simulink library "hose_pump_unit_v3"  (R2024a)
settings: Solver=VariableStepAuto  StartTime=0.0  StopTime=10.0  RelTol=1e-3
undefined symbols (not defined in the file): fiber_angle_alpha, fiber_angle_alpha_unstr, hose_pump_max_stretch, HP_spring_stiffness, HP_stretched_radius, HP_unstretched_length, HP_unstretched_radius, Lt, mu, regulator_set_pressure_PSI, Rt
libraries: fl_lib x5, nesl_utility x4, SimscapeFluids_lib x2
settings Model: Creator=Carson  LastModifiedBy=Carson

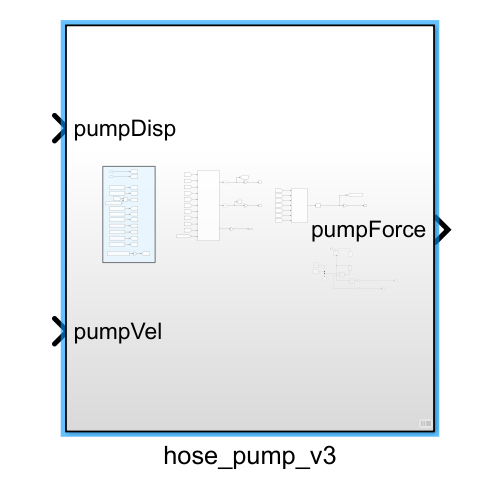
[thumbnail: Simulink's stored preview of the top-level diagram]
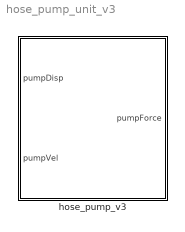
== system hose_pump_unit_v3 ==
  hose_pump_v3 : Subsystem

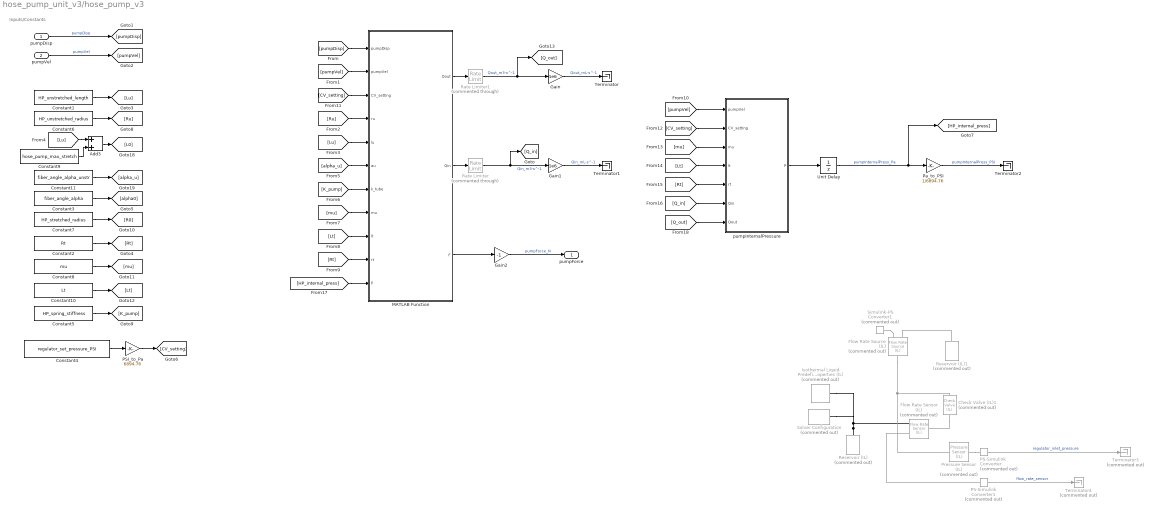
== system hose_pump_unit_v3/hose_pump_v3 ==
  note: Inputs/Constants
  pumpDisp : Inport
  pumpVel : Inport  Port=2
  Add3 : Sum
  Check Valve (IL)1 : SimscapeFluids_lib/Isothermal Liquid/Valves & Orifices/Directional Control Valves/Check Valve (IL)  Commented=on  opening_spec=fluids.isothermal_liquid.valves_orifices.enum.PressureOpeningSpec.Linear  pressure_control_spec=fluids.isothermal_liquid.valves_orifices.enum.pressure_control_spec.dp  p_crack_differential=regulator_set_pressure_PSI psi  p_crack_gauge=0.1 MPa  press_max_differential=regulator_set_pressure_PSI+1 psi  press_max_gauge=0.2 MPa  area_max=1e-4 m^2  area_leak=1e-10 m^2  p_diff_TLU=[0.01 : 0.01 : 0.1] MPa  valve_area_TLU=[1e-10, 1e-05, 2e-05, 3e-05, 4e-05, 5e-05, 6e-05, 7.5e-05, 8.5e-05, .0001] m^2  vol_flow_TLU=[.000358, .045, .11, .191, .284, .39, .505, .63, .764, .905] .* 1e-3 m^3/s  area=inf m^2  Cd=0.64  Re_c=150  smoothing_factor=0.01  pressure_recovery=false  opening_dynamics=false  tau=0.1 s  enable_faults=simscape.enum.onoff.off  fault_action=fluids.enum.FaultOpening.Closed
      settings: InternalSimscapePortConfiguration="{\"Bottom\":[],\"Left\":[{\"id\":\"A\",\"label\":\"A\",\"type\":\"foundation.isothermal_liquid.isothermal_liquid\"}],\"Right\":[{\"id\":\"B\",\"label\":\"B\",\"type\":\"foundation.isothermal_liquid.isothermal_liquid\"}],\"Top\":[]}"
  Constant1 : Constant  Value=HP_unstretched_length
  Constant10 : Constant  Value=Lt
  Constant11 : Constant  Value=fiber_angle_alpha_unstr
  Constant2 : Constant  Value=Rt
  Constant3 : Constant  Value=fiber_angle_alpha
  Constant4 : Constant  Value=regulator_set_pressure_PSI
  Constant5 : Constant  Value=HP_spring_stiffness
  Constant6 : Constant  Value=HP_unstretched_radius
  Constant7 : Constant  Value=HP_stretched_radius
  Constant8 : Constant  Value=mu
  Constant9 : Constant  Value=hose_pump_max_stretch
  Flow Rate Sensor (IL) : fl_lib/Isothermal Liquid/Sensors/Flow Rate Sensor (IL)  Commented=on  sensor_type=foundation.enum.mass_volumetric_sensor.volumetric
      settings: InternalSimscapePortConfiguration="{\"Bottom\":[],\"Left\":[{\"id\":\"A\",\"label\":\"A\",\"type\":\"foundation.isothermal_liquid.isothermal_liquid\"}],\"Right\":[{\"id\":\"B\",\"label\":\"B\",\"type\":\"foundation.isothermal_liquid.isothermal_liquid\"},{\"id\":\"V\",\"label\":\"V\",\"type\":\"output\"}],\"Top\":[]}"
  Flow Rate Source (IL) : fl_lib/Isothermal Liquid/Sources/Flow Rate Source (IL)  Commented=on  source_type=foundation.enum.constant_controlled.controlled  flow_type=foundation.enum.mass_volumetric_flow.volumetric  mass_flow=0 kg/s  volumetric_flow=0 m^3/s
      settings: InternalSimscapePortConfiguration="{\"Bottom\":[],\"Left\":[{\"id\":\"A\",\"label\":\"A\",\"type\":\"foundation.isothermal_liquid.isothermal_liquid\"},{\"id\":\"V\",\"label\":\"V\",\"type\":\"input\"}],\"Right\":[{\"id\":\"B\",\"label\":\"B\",\"type\":\"foundation.isothermal_liquid.isothermal_liquid\"}],\"Top\":[]}"
  Gain : Gain  Gain=1e6
  Gain1 : Gain  Gain=1e6
  Gain2 : Gain  Gain=-1
  Isothermal Liquid Predefined Properties (IL) : SimscapeFluids_lib/Isothermal Liquid/Utilities/Isothermal Liquid Predefined Properties (IL)  Commented=on  fluid_list=fluids.isothermal_liquid.utilities.enum.isothermal_liquid_fluid_list.water  concentration_param_EG=fluids.isothermal_liquid.utilities.enum.isothermal_liquid_concentration.volume_fraction  concentration_param_PG=fluids.isothermal_liquid.utilities.enum.isothermal_liquid_concentration.volume_fraction  c_mass_SW=3.5e-3  c_mass_EG=0.1  c_mass_PG=0.1  c_mass_GL=0.1  c_vol_EG=0.1  c_vol_PG=0.1  beta_L_atm_EG=2.1791 GPa  beta_L_atm_PG=2.1791 GPa  beta_L_atm_GL=2.1791 GPa  p_min_EG=0.01 MPa  p_min_PG=0.01 MPa  p_min_GL=0.01 MPa  T=293.15 K  derate_coeff=1  p_atm=0.101325 MPa  properties_range_check=simscape.enum.assert.action.warn  air_fraction=0  polytropic_index=1.0  rho_g_atm=1.225 kg/m^3  air_dissolution_model=false  p_crit=3 MPa
      settings: InternalSimscapePortConfiguration="{\"Bottom\":[],\"Left\":[],\"Right\":[{\"id\":\"A\",\"label\":\"\",\"type\":\"foundation.isothermal_liquid.isothermal_liquid\"}],\"Top\":[]}"
  MATLAB Function : MATLAB Function  TreatAsAtomicUnit=on
  PS-Simulink Converter : nesl_utility/PS-Simulink Converter  Commented=on  PhysicalDomain=network_engine_domain  SubClassName=ps_output  LeftPortType=input  RightPortType=output  PseudoPeriodic=off  Frequencies=[]  VectorFormat=inherit  Unit=Pa  AffineConversion=off
  PS-Simulink Converter1 : nesl_utility/PS-Simulink Converter  Commented=on  PhysicalDomain=network_engine_domain  SubClassName=ps_output  LeftPortType=input  RightPortType=output  PseudoPeriodic=off  Frequencies=[]  VectorFormat=inherit  Unit=m^3/s  AffineConversion=off
  PSI_to_Pa : Gain  Gain=6894.76
  Pa_to_PSI : Gain  Gain=1/6894.76
  Pressure Sensor (IL) : fl_lib/Isothermal Liquid/Sensors/Pressure Sensor (IL)  Commented=on  pressure_measure=foundation.enum.pressure_measure.gauge
      settings: InternalSimscapePortConfiguration="{\"Bottom\":[],\"Left\":[{\"id\":\"A\",\"label\":\"A\",\"type\":\"foundation.isothermal_liquid.isothermal_liquid\"}],\"Right\":[{\"id\":\"Pg\",\"label\":\"Pg\",\"type\":\"output\"}],\"Top\":[]}"
  Rate Limiter : RateLimiter  Commented=through  RisingSlewLimit=1e-3  FallingSlewLimit=-1e-3  SampleTimeMode=inherited
  Rate Limiter1 : RateLimiter  Commented=through  RisingSlewLimit=1e-3  FallingSlewLimit=-1e-3  SampleTimeMode=inherited
  Reservoir (IL) : fl_lib/Isothermal Liquid/Elements/Reservoir (IL)  Commented=on  reservoir_type=foundation.enum.constant_controlled.constant  pressure_spec=foundation.enum.pressure_spec.atmospheric  reservoir_pressure=0.101325 MPa
  Reservoir (IL)1 : fl_lib/Isothermal Liquid/Elements/Reservoir (IL)  Commented=on  reservoir_type=foundation.enum.constant_controlled.constant  pressure_spec=foundation.enum.pressure_spec.atmospheric  reservoir_pressure=0.101325 MPa
  Simulink-PS Converter1 : nesl_utility/Simulink-PS Converter  Commented=on  PhysicalDomain=network_engine_domain  SubClassName=ps_input  LeftPortType=input  RightPortType=output  PseudoPeriodic=off  Frequencies=[]  NoiseDistribution=none  NoiseParameters=[]  Unit=m^3/s  AffineConversion=off  FilteringAndDerivatives=zero  SimscapeFilterOrder=1  InputFilterTimeConstant=0.001  UdotUserProvided=0
  Solver Configuration : nesl_utility/Solver Configuration  Commented=on  PhysicalDomain=network_engine_domain  SubClassName=solver  LeftPortType=input  RightPortType=generic  Tones=[]  Harmonics=[]  SimulateNoise=off  Profile=off  UseLocalSampling=off  EnableSwitchedLinearOptims=on  FrequencyDomain=off  UseCCode=off  RelTol=0.001  AbsTol=1e-06  MinStep=1e-09  ToWorkspace=off  RevertToSquareIcSolve=off  NumHomotopyIterations=100  PhasorMode=off  PhasorModeNumHarmonics=1  ConsistencySolver=NEWTON_XTOL_AFTER_FTOL  IndexReductionMethod=DerivativeReplacement  DoDC=on  ResidualTolerance=1e-09  ConsistencyTolSource=GLOBAL  ConsistencyAbsTol=0.001  ConsistencyRelTol=0.001  ConsistencyTolFactor=0.001  UseLocalSolver=on  LocalSolverChoice=NE_BACKWARD_EULER_ADVANCER  ResolveIndetEquations=on  FunctionEvalNumThread=1  LocalSolverSampleTime=simu.dt  DoFixedCost=off  MaxNonlinIter=3  MaxModeIter=2  ComputeImpulses=off  ImpulseIterations=2  LinearAlgebra=auto  LinearAlgebraNumThread=0  EquationFormulation=NE_TIME_EF  DelaysMemoryBudget=1024  AutomaticFiltering=off  FilteringTimeConstant=0.001  PartitionStorageMethod=AS_NEEDED  PartitionMemoryBudget=1024  PartitionMethod=FAST  MultibodyUseLocalSolver=off  MultibodyLocalSolverChoice=ODE1  MultibodyLocalSolverSampleTime=0.001
  Terminator : Terminator
  Terminator1 : Terminator
  Terminator2 : Terminator
  Terminator3 : Terminator  Commented=on
  Terminator4 : Terminator  Commented=on
  Unit Delay : UnitDelay  SampleTime=-1  HasFrameUpgradeWarning=on
  pumpInternalPressure : MATLAB Function  TreatAsAtomicUnit=on
  pumpForce : Outport
  wires:
  Constant3/1 -> [alpha0]
  Constant2/1 -> [Rt]
  Constant1/1 -> [Lu]
  Constant5/1 -> [K_pump]
  Constant9/1 -> Add3/2
  [Lu] -> Add3/1
  Add3/1 -> [L0]
  Constant11/1 -> [alpha_u]
  pumpDisp/1 -> [pumpDisp]  "pumpDisp"
  pumpVel/1 -> [pumpVel]  "pumpVel"
  Constant6/1 -> [Ru]
  Constant7/1 -> [R0]
  Constant8/1 -> [mu]
  Constant10/1 -> [Lt]
  [pumpDisp] -> MATLAB Function/1(pumpDisp)
  [pumpVel] -> MATLAB Function/2(pumpVel)
  [Ru] -> MATLAB Function/4(ru)
  [Lu] -> MATLAB Function/5(lu)
  [alpha_u] -> MATLAB Function/6(au)
  [K_pump] -> MATLAB Function/7(k_tube)
  [mu] -> MATLAB Function/8(mu)
  [Lt] -> MATLAB Function/9(lt)
  [Rt] -> MATLAB Function/10(rt)
  Rate Limiter1/1 -> [Q_out], Gain/1  "Qout_m3-s^-1"
  Rate Limiter/1 -> [Q_in], Gain1/1  "Qin_m3-s^-1"
  Unit Delay/1 -> [HP_internal_press], Pa_to_PSI/1  "pumpInternalPress_Pa"
  [CV_setting] -> MATLAB Function/3(CV_setting)
  Gain/1 -> Terminator/1  "Qout_mL-s^-1"
  Gain1/1 -> Terminator1/1  "Qin_mL-s^-1"
  Pa_to_PSI/1 -> Terminator2/1  "pumpInternalPress_PSI"
  Gain2/1 -> pumpForce/1  "pumpForce_N"
  MATLAB Function/3(F) -> Gain2/1
  [pumpVel] -> pumpInternalPressure/1(pumpVel)
  Constant4/1 -> PSI_to_Pa/1
  PSI_to_Pa/1 -> [CV_setting]
  [CV_setting] -> pumpInternalPressure/2(CV_setting)
  [mu] -> pumpInternalPressure/3(mu)
  [Lt] -> pumpInternalPressure/4(lt)
  [Rt] -> pumpInternalPressure/5(rt)
  [Q_in] -> pumpInternalPressure/6(Qin)
  [HP_internal_press] -> MATLAB Function/11(P)
  pumpInternalPressure/1(P) -> Unit Delay/1
  PS-Simulink Converter/1 -> Terminator3/1  "regulator_inlet_pressure"
  PS-Simulink Converter1/1 -> Terminator4/1  "flow_rate_sensor"
  [Q_out] -> pumpInternalPressure/7(Qout)
  MATLAB Function/2(Qin) -> Rate Limiter/1
  MATLAB Function/1(Qout) -> Rate Limiter1/1
  connections:
  Reservoir (IL)/LConn1 -- Flow Rate Sensor (IL)/RConn1 -- Solver Configuration/RConn1 -- Isothermal Liquid Predefined Properties (IL)/RConn1
  Flow Rate Source (IL)/RConn1 -- Check Valve (IL)1/LConn1 -- Pressure Sensor (IL)/LConn1
  PS-Simulink Converter1/LConn1 -- Flow Rate Sensor (IL)/RConn2
  Reservoir (IL)1/LConn1 -- Flow Rate Source (IL)/LConn1
  Simulink-PS Converter1/RConn1 -- Flow Rate Source (IL)/LConn2
  Check Valve (IL)1/RConn1 -- Flow Rate Sensor (IL)/LConn1
  Pressure Sensor (IL)/RConn1 -- PS-Simulink Converter/LConn1

== matlab function hose_pump_unit_v3/hose_pump_v3/MATLAB Function ==
  data: pumpDisp input; pumpVel input; CV_setting input; Qout output; ru input; lu input; au input; k_tube input; mu input; lt input; rt input; Qin output; F output; P input
function [Qout, Qin, F] = pumpDisplacementCalcs(pumpDisp, pumpVel, CV_setting, ru, lu, au, k_tube, mu, lt, rt, P)

if pumpVel > 0 % pumping water out
    % P = CV_setting; % assume internal pressure immediately rises to check valve set pressure
    % F = pi * ru^2 * P * (3 * (pumpDisp/lu+1)^2 / (tan(au))^2 - 1/sin(au)^2) + k_tube*pumpDisp;
    Qout = -pi * ru^2 * (1/sin(au)^2 - 3 * (pumpDisp/lu+1)^2 / (tan(au))^2) * pumpVel;
    Qin = 0;
else
    % F = k_tube*pumpDisp;
    Qin = pi * ru^2 * (1/sin(au)^2 - 3 * (pumpDisp/lu+1)^2 / (tan(au))^2) * pumpVel;
    Qout = 0;
    % P = -8*mu*lt/(pi*rt^4)*Qin;
end

F = pi * ru^2 * max([P, 0]) * (3 * (pumpDisp/lu+1)^2 / (tan(au))^2 - 1/sin(au)^2) + k_tube*pumpDisp;

== matlab function hose_pump_unit_v3/hose_pump_v3/pumpInternalPressure ==
  data: pumpVel input; CV_setting input; mu input; lt input; rt input; Qin input; P output; Qout input
function P  = pumpInternalPressure(pumpVel, CV_setting, mu, lt, rt, Qin, Qout)

if Qout > 0 % pumping water out
    P = CV_setting;
    %debug = [8*mu*lt/(pi*rt^4)*Qout, CV_setting];
else
    P = -8*mu*lt/(pi*rt^4)*Qin;
end
